simulink library "Environment_UL"  (R2019a)
settings: Solver=VariableStepAuto  StartTime=0.0  StopTime=10.0  RelTol=1e-3
undefined symbols (not defined in the file): ENV, Motor
libraries: simulink x2
settings Model: Creator=John Jr  LastModifiedBy=John Jr

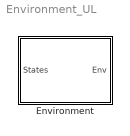
== system Environment_UL ==
  Environment : Subsystem  mask{g=ENV.g, rho_b=ENV.rho_b, z_0=ENV.z_0, T=ENV.T, M=ENV.M, R=ENV.R, v_w0=ENV.v_w0, v_wf=ENV.v_wf}
      mask prompts: g "Gravitational acceleration [m/s^2]"; rho_b "Air density at sea level [kg/m^3]"; z_0 "Initial altitude above sea level [m]"; T "Air temperature [K]"; M "Molar mass of air [kg/mol]"; R "Gas constant [Nm/(mol.K)]"; v_w0 "Wind speed at ground level [m/s]"; v_wf "Wind speed at 5000 ft [m/s]"
      mask DialogControl DescGroupVar Prompt: Environment
      mask DialogControl DescTextVar Prompt: This block models the air density and wind speed as a function of altitude.
      mask DialogControl Control2 Prompt: Air Density Parameters:
      mask DialogControl Control3 Prompt: Wind Speed Parameters:
      mask Display:
      | patch([0 1 1 0], [0 0 1 1],[.8 1 1])
      | 
      | port_label('input',1,'\fontname{Cambria Math}States','texmode','on')
      | 
      | port_label('output',1,'\fontname{Cambria Math}Env','texmode','on')

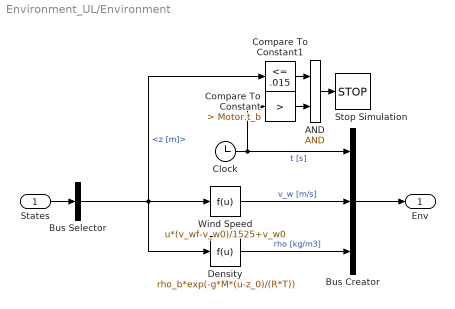
== system Environment_UL/Environment ==
  States : Inport
  AND : Logic  IconShape=distinctive  AllPortsSameDT=off  OutDataTypeStr=boolean
  Bus Creator : BusCreator  Inputs=3
  Bus Selector : BusSelector  OutputSignals=Z.z [m]
  Clock : Clock
  Compare To Constant : simulink/Logic and Bit Operations/Compare To Constant  relop=>  const=Motor.t_b  OutDataTypeStr=boolean
  Compare To Constant1 : simulink/Logic and Bit Operations/Compare To Constant  relop=<=  const=.015  OutDataTypeStr=boolean
  Density : Fcn  Expr=rho_b*exp(-g*M*(u-z_0)/(R*T))
  Stop Simulation : Stop
  Wind Speed : Fcn  Expr=u*(v_wf-v_w0)/1525+v_w0
  Env : Outport
  wires:
  Bus Selector/1 -> Compare To Constant1/1, Wind Speed/1, Density/1  "<z [m]>"
  Density/1 -> Bus Creator/3  "rho [kg/m3]"
  Wind Speed/1 -> Bus Creator/2  "v_w [m/s]"
  States/1 -> Bus Selector/1
  Bus Creator/1 -> Env/1
  Clock/1 -> Compare To Constant/1, Bus Creator/1  "t [s]"
  AND/1 -> Stop Simulation/1
  Compare To Constant/1 -> AND/2
  Compare To Constant1/1 -> AND/1
